simulink model "EPT"  (R2019b)
settings: Solver=FixedStepDiscrete  StartTime=0.0  StopTime=5  FixedStep=0.005  RelTol=1e-3  EnableMultiTasking=on
PreLoadFcn:
  | try, model_open; catch, disp('Error occurred while executing model pre-load callback: model_open.m'); disp('Please assure that the MATLAB working directory is set to the model directory before opening.'); end
InitFcn:
  | try, model_open; catch, end
undefined symbols (not defined in the file or in its folder): Bridge, GCM, H, ln, raptor_get_param_eval, raptor_get_safe_string, raptor_xcp_function
libraries: Raptor_lib x2810, simulink x374, hdlsllib x19
(part 7 of 45)

== system EPT/I//O/Output/DualLED_Half_Bridge ==
  note: H3
  note: H1
  Data Type Conversion : DataTypeConversion
  Data Type Conversion3 : DataTypeConversion
  Gain : Gain  Gain=100
  Gain3 : Gain  Gain=100
  raptor_adjustment1 : Raptor_lib/Data Storage/raptor_adjustment  paramName='A43_A44_HalfBridge_Brake'  nameSource=Parameter  initValue=0.00  dataType=boolean  storage=Calibration  calDispType=Number  calEnum={'False', 'True'}  calGain=1.0  calOffset=0.0  calMax=inf  calMin=-inf  calFormat='-1'  calUnit=''  calHelp=''  calAccess=1  calFunction=raptor_xcp_function(gcb)  calDispHeaders=off  calColHeaders={'Col1' 'Col2' 'Col3'}  calRowHeaders={'Row1' 'Row2' 'Row3'}
      settings: SourceProductName=Raptor
  raptor_adjustment2 : Raptor_lib/Data Storage/raptor_adjustment  paramName='Cal_HalfBridge3_Freq'  nameSource=Parameter  initValue=1000  dataType=uint16  storage=Calibration  calDispType=Number  calEnum={'False', 'True'}  calGain=1.0  calOffset=0.0  calMax=inf  calMin=-inf  calFormat='-1'  calUnit=''  calHelp=''  calAccess=1  calFunction=raptor_xcp_function(gcb)  calDispHeaders=off  calColHeaders={'Col1' 'Col2' 'Col3'}  calRowHeaders={'Row1' 'Row2' 'Row3'}
      settings: SourceProductName=Raptor
  raptor_adjustment3 : Raptor_lib/Data Storage/raptor_adjustment  paramName='Cal_HalfBridge3_En'  nameSource=Parameter  initValue=1  dataType=boolean  storage=Calibration  calDispType=Number  calEnum={'False', 'True'}  calGain=1.0  calOffset=0.0  calMax=inf  calMin=-inf  calFormat='-1'  calUnit=''  calHelp=''  calAccess=1  calFunction=raptor_xcp_function(gcb)  calDispHeaders=off  calColHeaders={'Col1' 'Col2' 'Col3'}  calRowHeaders={'Row1' 'Row2' 'Row3'}
      settings: SourceProductName=Raptor
  raptor_adjustment4 : Raptor_lib/Data Storage/raptor_adjustment  paramName='A66_A67_HalfBridge_Brake'  nameSource=Parameter  initValue=0.00  dataType=boolean  storage=Calibration  calDispType=Number  calEnum={'False', 'True'}  calGain=1.0  calOffset=0.0  calMax=inf  calMin=-inf  calFormat='-1'  calUnit=''  calHelp=''  calAccess=1  calFunction=raptor_xcp_function(gcb)  calDispHeaders=off  calColHeaders={'Col1' 'Col2' 'Col3'}  calRowHeaders={'Row1' 'Row2' 'Row3'}
      settings: SourceProductName=Raptor
  raptor_adjustment5 : Raptor_lib/Data Storage/raptor_adjustment  paramName='Cal_HalfBridge1_Freq'  nameSource=Parameter  initValue=1000  dataType=uint16  storage=Calibration  calDispType=Number  calEnum={'False', 'True'}  calGain=1.0  calOffset=0.0  calMax=inf  calMin=-inf  calFormat='-1'  calUnit=''  calHelp=''  calAccess=1  calFunction=raptor_xcp_function(gcb)  calDispHeaders=off  calColHeaders={'Col1' 'Col2' 'Col3'}  calRowHeaders={'Row1' 'Row2' 'Row3'}
      settings: SourceProductName=Raptor
  raptor_adjustment6 : Raptor_lib/Data Storage/raptor_adjustment  paramName='Cal_HalfBridge1_En'  nameSource=Parameter  initValue=1  dataType=boolean  storage=Calibration  calDispType=Number  calEnum={'False', 'True'}  calGain=1.0  calOffset=0.0  calMax=inf  calMin=-inf  calFormat='-1'  calUnit=''  calHelp=''  calAccess=1  calFunction=raptor_xcp_function(gcb)  calDispHeaders=off  calColHeaders={'Col1' 'Col2' 'Col3'}  calRowHeaders={'Row1' 'Row2' 'Row3'}
      settings: SourceProductName=Raptor
  raptor_data_read : Raptor_lib/Data Storage/raptor_data_read  dataName='LED_Duty'  dataShape=Scalar  idxSource=Input  idxRow=1  idxCol=1
      settings: SourceProductName=Raptor
  raptor_hbridge_out : Raptor_lib/Input & Output/raptor_hbridge_out  resourceValues=OUTPUT50_51|OUTPUT52_53|OUTPUT54_55|(None)  resource=OUTPUT54_55  outError=0  driverTypeValues=H-Bridge  driverType=H-Bridge
      settings: SourceProductName=Raptor
  raptor_hbridge_out1 : Raptor_lib/Input & Output/raptor_hbridge_out  resourceValues=OUTPUT50_51|OUTPUT52_53|OUTPUT54_55|(None)  resource=OUTPUT50_51  outError=0  driverTypeValues=H-Bridge  driverType=H-Bridge
      settings: SourceProductName=Raptor
  wires:
  raptor_adjustment1/1 -> raptor_hbridge_out/2
  raptor_data_read/1 -> raptor_hbridge_out1/3, raptor_hbridge_out/3
  Gain/1 -> Data Type Conversion/1
  Data Type Conversion/1 -> raptor_hbridge_out/4
  raptor_adjustment3/1 -> raptor_hbridge_out/1
  raptor_adjustment2/1 -> Gain/1
  raptor_adjustment4/1 -> raptor_hbridge_out1/2
  raptor_adjustment5/1 -> Gain3/1
  Data Type Conversion3/1 -> raptor_hbridge_out1/4
  Gain3/1 -> Data Type Conversion3/1
  raptor_adjustment6/1 -> raptor_hbridge_out1/1

== system EPT/I//O/Output/Lamp_Sound ==
  raptor_adjustment : Raptor_lib/Data Storage/raptor_adjustment  paramName='A01_LSD_EW_Sound1'  nameSource=Parameter  initValue=0.00  dataType=boolean  storage=Calibration  calDispType=Number  calEnum={'False', 'True'}  calGain=1.0  calOffset=0.0  calMax=inf  calMin=-inf  calFormat='-1'  calUnit=''  calHelp=''  calAccess=1  calFunction=raptor_xcp_function(gcb)  calDispHeaders=off  calColHeaders={'Col1' 'Col2' 'Col3'}  calRowHeaders={'Row1' 'Row2' 'Row3'}
      settings: SourceProductName=Raptor
  raptor_adjustment3 : Raptor_lib/Data Storage/raptor_adjustment  paramName='A54_EW_Lamp_Sound3'  nameSource=Parameter  initValue=0.00  dataType=boolean  storage=Calibration  calDispType=Number  calEnum={'False', 'True'}  calGain=1.0  calOffset=0.0  calMax=inf  calMin=-inf  calFormat='-1'  calUnit=''  calHelp=''  calAccess=1  calFunction=raptor_xcp_function(gcb)  calDispHeaders=off  calColHeaders={'Col1' 'Col2' 'Col3'}  calRowHeaders={'Row1' 'Row2' 'Row3'}
      settings: SourceProductName=Raptor
  raptor_digital_out : Raptor_lib/Input & Output/raptor_digital_out  resourceValues=OUTPUT1|OUTPUT2|OUTPUT3|OUTPUT4|OUTPUT5|OUTPUT6|OUTPUT7|OUTPUT8|OUTPUT9|OUTPUT10|OUTPUT11|OUTPUT12|OUTPUT21|OUTPUT22|OUTPUT23|OUTPUT24|OUTPUT25|OUTPUT26|OUTPUT27|OUTPUT28|OUTPUT29|OUTPUT30|OUTPUT31|OUTPUT32|OUTPUT33|OUTPUT34|OUTPUT35|OUTPUT36|OUTPUT37|OUTPUT38|OUTPUT39|OUTPUT40|OUTPUT41|OUTPUT42|OUTPUT43|OUTPUT44|OUTPUT45|OUTPUT46|OUTPUT47|OUTPUT48|OUTPUT49|POWER_HOLD|(None)  resource=OUTPUT25  driverTypeValues=Low Side  driverType=Low Side
      settings: SourceProductName=Raptor
  raptor_digital_out3 : Raptor_lib/Input & Output/raptor_digital_out  resourceValues=OUTPUT1|OUTPUT2|OUTPUT3|OUTPUT4|OUTPUT5|OUTPUT6|OUTPUT7|OUTPUT8|OUTPUT9|OUTPUT10|OUTPUT11|OUTPUT12|OUTPUT21|OUTPUT22|OUTPUT23|OUTPUT24|OUTPUT25|OUTPUT26|OUTPUT27|OUTPUT28|OUTPUT29|OUTPUT30|OUTPUT31|OUTPUT32|OUTPUT33|OUTPUT34|OUTPUT35|OUTPUT36|OUTPUT37|OUTPUT38|OUTPUT39|OUTPUT40|OUTPUT41|OUTPUT42|OUTPUT43|OUTPUT44|OUTPUT45|OUTPUT46|OUTPUT47|OUTPUT48|OUTPUT49|POWER_HOLD|(None)  resource=OUTPUT5  driverTypeValues=Low Side  driverType=Low Side
      settings: SourceProductName=Raptor
  wires:
  raptor_adjustment3/1 -> raptor_digital_out3/1
  raptor_adjustment/1 -> raptor_digital_out/1

== system EPT/I//O/Output/RelayBox ==
  Bitwe Operator{2..7} (6 alike) : simulink/Logic and Bit Operations/Bitwise Operator  logicop=OR  UseBitMask=off  NumInputPorts=2  BitMask=bin2dec('11011001')  BitMaskRealWorld=Stored Integer
  raptor_adjustment : Raptor_lib/Data Storage/raptor_adjustment  paramName='K12_LSD_Relay_HV_Body'  nameSource=Parameter  initValue=0.00  dataType=boolean  storage=Calibration  calDispType=Number  calEnum={'False', 'True'}  calGain=1.0  calOffset=0.0  calMax=inf  calMin=-inf  calFormat='-1'  calUnit=''  calHelp=''  calAccess=1  calFunction=raptor_xcp_function(gcb)  calDispHeaders=off  calColHeaders={'Col1' 'Col2' 'Col3'}  calRowHeaders={'Row1' 'Row2' 'Row3'}
      settings: SourceProductName=Raptor
  raptor_adjustment2 : Raptor_lib/Data Storage/raptor_adjustment  paramName='K20_LSD_Relay_DCDC_12V'  nameSource=Parameter  initValue=0.00  dataType=boolean  storage=Calibration  calDispType=Number  calEnum={'False', 'True'}  calGain=1.0  calOffset=0.0  calMax=inf  calMin=-inf  calFormat='-1'  calUnit=''  calHelp=''  calAccess=1  calFunction=raptor_xcp_function(gcb)  calDispHeaders=off  calColHeaders={'Col1' 'Col2' 'Col3'}  calRowHeaders={'Row1' 'Row2' 'Row3'}
      settings: SourceProductName=Raptor
  raptor_adjustment3 : Raptor_lib/Data Storage/raptor_adjustment  paramName='K36_LSD_Relay_CHG_OBC'  nameSource=Parameter  initValue=0.00  dataType=boolean  storage=Calibration  calDispType=Number  calEnum={'False', 'True'}  calGain=1.0  calOffset=0.0  calMax=inf  calMin=-inf  calFormat='-1'  calUnit=''  calHelp=''  calAccess=1  calFunction=raptor_xcp_function(gcb)  calDispHeaders=off  calColHeaders={'Col1' 'Col2' 'Col3'}  calRowHeaders={'Row1' 'Row2' 'Row3'}
      settings: SourceProductName=Raptor
  raptor_adjustment4 : Raptor_lib/Data Storage/raptor_adjustment  paramName='K38_LSD_Relay_BMS_OBU'  nameSource=Parameter  initValue=0.00  dataType=boolean  storage=Calibration  calDispType=Number  calEnum={'False', 'True'}  calGain=1.0  calOffset=0.0  calMax=inf  calMin=-inf  calFormat='-1'  calUnit=''  calHelp=''  calAccess=1  calFunction=raptor_xcp_function(gcb)  calDispHeaders=off  calColHeaders={'Col1' 'Col2' 'Col3'}  calRowHeaders={'Row1' 'Row2' 'Row3'}
      settings: SourceProductName=Raptor
  raptor_adjustment5 : Raptor_lib/Data Storage/raptor_adjustment  paramName='K39_LSD_Relay_MCU'  nameSource=Parameter  initValue=0.00  dataType=boolean  storage=Calibration  calDispType=Number  calEnum={'False', 'True'}  calGain=1.0  calOffset=0.0  calMax=inf  calMin=-inf  calFormat='-1'  calUnit=''  calHelp=''  calAccess=1  calFunction=raptor_xcp_function(gcb)  calDispHeaders=off  calColHeaders={'Col1' 'Col2' 'Col3'}  calRowHeaders={'Row1' 'Row2' 'Row3'}
      settings: SourceProductName=Raptor
  raptor_adjustment6 : Raptor_lib/Data Storage/raptor_adjustment  paramName='K56_LSD_Relay_BMS_SWU'  nameSource=Parameter  initValue=0.00  dataType=boolean  storage=Calibration  calDispType=Number  calEnum={'False', 'True'}  calGain=1.0  calOffset=0.0  calMax=inf  calMin=-inf  calFormat='-1'  calUnit=''  calHelp=''  calAccess=1  calFunction=raptor_xcp_function(gcb)  calDispHeaders=off  calColHeaders={'Col1' 'Col2' 'Col3'}  calRowHeaders={'Row1' 'Row2' 'Row3'}
      settings: SourceProductName=Raptor
  raptor_data_def : Raptor_lib/Data Storage/raptor_data_def  dataName='Relay_HV_Body'  initValue=0  dataType=boolean  storage=Volatile (RAM)  calVisible=on  calType=Measurement  calDispType=Number  calEnum={'False', 'True'}  calGain=1.0  calOffset=0  calMin=-inf  calMax=inf  calFormat='-1'  calUnit=''  calHelp=''  calAccess=1  calFunction=raptor_xcp_function(gcb)  calDispHeaders=off  calColHeaders={'Col1' 'Col2' 'Col3'}  calRowHeaders={'Row1' 'Row2' 'Row3'}
      settings: SourceProductName=Raptor
  raptor_data_def2 : Raptor_lib/Data Storage/raptor_data_def  dataName='Relay_DCDC_12V'  initValue=0  dataType=boolean  storage=Volatile (RAM)  calVisible=on  calType=Measurement  calDispType=Number  calEnum={'False', 'True'}  calGain=1.0  calOffset=0  calMin=-inf  calMax=inf  calFormat='-1'  calUnit=''  calHelp=''  calAccess=1  calFunction=raptor_xcp_function(gcb)  calDispHeaders=off  calColHeaders={'Col1' 'Col2' 'Col3'}  calRowHeaders={'Row1' 'Row2' 'Row3'}
      settings: SourceProductName=Raptor
  raptor_data_def3 : Raptor_lib/Data Storage/raptor_data_def  dataName='Relay_CHG_OBC'  initValue=0  dataType=boolean  storage=Volatile (RAM)  calVisible=on  calType=Measurement  calDispType=Number  calEnum={'False', 'True'}  calGain=1.0  calOffset=0  calMin=-inf  calMax=inf  calFormat='-1'  calUnit=''  calHelp=''  calAccess=1  calFunction=raptor_xcp_function(gcb)  calDispHeaders=off  calColHeaders={'Col1' 'Col2' 'Col3'}  calRowHeaders={'Row1' 'Row2' 'Row3'}
      settings: SourceProductName=Raptor
  raptor_data_def4 : Raptor_lib/Data Storage/raptor_data_def  dataName='Relay_BMS_OBU'  initValue=0  dataType=boolean  storage=Volatile (RAM)  calVisible=on  calType=Measurement  calDispType=Number  calEnum={'False', 'True'}  calGain=1.0  calOffset=0  calMin=-inf  calMax=inf  calFormat='-1'  calUnit=''  calHelp=''  calAccess=1  calFunction=raptor_xcp_function(gcb)  calDispHeaders=off  calColHeaders={'Col1' 'Col2' 'Col3'}  calRowHeaders={'Row1' 'Row2' 'Row3'}
      settings: SourceProductName=Raptor
  raptor_data_def5 : Raptor_lib/Data Storage/raptor_data_def  dataName='Relay_MCU'  initValue=0  dataType=boolean  storage=Volatile (RAM)  calVisible=on  calType=Measurement  calDispType=Number  calEnum={'False', 'True'}  calGain=1.0  calOffset=0  calMin=-inf  calMax=inf  calFormat='-1'  calUnit=''  calHelp=''  calAccess=1  calFunction=raptor_xcp_function(gcb)  calDispHeaders=off  calColHeaders={'Col1' 'Col2' 'Col3'}  calRowHeaders={'Row1' 'Row2' 'Row3'}
      settings: SourceProductName=Raptor
  raptor_data_def6 : Raptor_lib/Data Storage/raptor_data_def  dataName='Relay_BMS_SWU'  initValue=0  dataType=boolean  storage=Volatile (RAM)  calVisible=on  calType=Measurement  calDispType=Number  calEnum={'False', 'True'}  calGain=1.0  calOffset=0  calMin=-inf  calMax=inf  calFormat='-1'  calUnit=''  calHelp=''  calAccess=1  calFunction=raptor_xcp_function(gcb)  calDispHeaders=off  calColHeaders={'Col1' 'Col2' 'Col3'}  calRowHeaders={'Row1' 'Row2' 'Row3'}
      settings: SourceProductName=Raptor
  raptor_data_read : Raptor_lib/Data Storage/raptor_data_read  dataName='Relay_BMS_OBU'  dataShape=Scalar  idxSource=Input  idxRow=1  idxCol=1
      settings: SourceProductName=Raptor
  raptor_data_read1 : Raptor_lib/Data Storage/raptor_data_read  dataName='Relay_MCU'  dataShape=Scalar  idxSource=Input  idxRow=1  idxCol=1
      settings: SourceProductName=Raptor
  raptor_data_read2 : Raptor_lib/Data Storage/raptor_data_read  dataName='Relay_BMS_SWU'  dataShape=Scalar  idxSource=Input  idxRow=1  idxCol=1
      settings: SourceProductName=Raptor
  raptor_data_read4 : Raptor_lib/Data Storage/raptor_data_read  dataName='Relay_CHG_OBC'  dataShape=Scalar  idxSource=Input  idxRow=1  idxCol=1
      settings: SourceProductName=Raptor
  raptor_data_read5 : Raptor_lib/Data Storage/raptor_data_read  dataName='Relay_DCDC_12V'  dataShape=Scalar  idxSource=Input  idxRow=1  idxCol=1
      settings: SourceProductName=Raptor
  raptor_data_read7 : Raptor_lib/Data Storage/raptor_data_read  dataName='Relay_HV_Body'  dataShape=Scalar  idxSource=Input  idxRow=1  idxCol=1
      settings: SourceProductName=Raptor
  raptor_digital_out : Raptor_lib/Input & Output/raptor_digital_out  resourceValues=OUTPUT1|OUTPUT2|OUTPUT3|OUTPUT4|OUTPUT5|OUTPUT6|OUTPUT7|OUTPUT8|OUTPUT9|OUTPUT10|OUTPUT11|OUTPUT12|OUTPUT21|OUTPUT22|OUTPUT23|OUTPUT24|OUTPUT25|OUTPUT26|OUTPUT27|OUTPUT28|OUTPUT29|OUTPUT30|OUTPUT31|OUTPUT32|OUTPUT33|OUTPUT34|OUTPUT35|OUTPUT36|OUTPUT37|OUTPUT38|OUTPUT39|OUTPUT40|OUTPUT41|OUTPUT42|OUTPUT43|OUTPUT44|OUTPUT45|OUTPUT46|OUTPUT47|OUTPUT48|OUTPUT49|POWER_HOLD|(None)  resource=OUTPUT33  driverTypeValues=Low Side  driverType=Low Side
      settings: SourceProductName=Raptor
  raptor_digital_out2 : Raptor_lib/Input & Output/raptor_digital_out  resourceValues=OUTPUT1|OUTPUT2|OUTPUT3|OUTPUT4|OUTPUT5|OUTPUT6|OUTPUT7|OUTPUT8|OUTPUT9|OUTPUT10|OUTPUT11|OUTPUT12|OUTPUT21|OUTPUT22|OUTPUT23|OUTPUT24|OUTPUT25|OUTPUT26|OUTPUT27|OUTPUT28|OUTPUT29|OUTPUT30|OUTPUT31|OUTPUT32|OUTPUT33|OUTPUT34|OUTPUT35|OUTPUT36|OUTPUT37|OUTPUT38|OUTPUT39|OUTPUT40|OUTPUT41|OUTPUT42|OUTPUT43|OUTPUT44|OUTPUT45|OUTPUT46|OUTPUT47|OUTPUT48|OUTPUT49|POWER_HOLD|(None)  resource=OUTPUT35  driverTypeValues=Low Side  driverType=Low Side
      settings: SourceProductName=Raptor
  raptor_digital_out3 : Raptor_lib/Input & Output/raptor_digital_out  resourceValues=OUTPUT1|OUTPUT2|OUTPUT3|OUTPUT4|OUTPUT5|OUTPUT6|OUTPUT7|OUTPUT8|OUTPUT9|OUTPUT10|OUTPUT11|OUTPUT12|OUTPUT21|OUTPUT22|OUTPUT23|OUTPUT24|OUTPUT25|OUTPUT26|OUTPUT27|OUTPUT28|OUTPUT29|OUTPUT30|OUTPUT31|OUTPUT32|OUTPUT33|OUTPUT34|OUTPUT35|OUTPUT36|OUTPUT37|OUTPUT38|OUTPUT39|OUTPUT40|OUTPUT41|OUTPUT42|OUTPUT43|OUTPUT44|OUTPUT45|OUTPUT46|OUTPUT47|OUTPUT48|OUTPUT49|POWER_HOLD|(None)  resource=OUTPUT37  driverTypeValues=Low Side  driverType=Low Side
      settings: SourceProductName=Raptor
  raptor_digital_out4 : Raptor_lib/Input & Output/raptor_digital_out  resourceValues=OUTPUT1|OUTPUT2|OUTPUT3|OUTPUT4|OUTPUT5|OUTPUT6|OUTPUT7|OUTPUT8|OUTPUT9|OUTPUT10|OUTPUT11|OUTPUT12|OUTPUT21|OUTPUT22|OUTPUT23|OUTPUT24|OUTPUT25|OUTPUT26|OUTPUT27|OUTPUT28|OUTPUT29|OUTPUT30|OUTPUT31|OUTPUT32|OUTPUT33|OUTPUT34|OUTPUT35|OUTPUT36|OUTPUT37|OUTPUT38|OUTPUT39|OUTPUT40|OUTPUT41|OUTPUT42|OUTPUT43|OUTPUT44|OUTPUT45|OUTPUT46|OUTPUT47|OUTPUT48|OUTPUT49|POWER_HOLD|(None)  resource=OUTPUT38  driverTypeValues=Low Side  driverType=Low Side
      settings: SourceProductName=Raptor
  raptor_digital_out5 : Raptor_lib/Input & Output/raptor_digital_out  resourceValues=OUTPUT1|OUTPUT2|OUTPUT3|OUTPUT4|OUTPUT5|OUTPUT6|OUTPUT7|OUTPUT8|OUTPUT9|OUTPUT10|OUTPUT11|OUTPUT12|OUTPUT21|OUTPUT22|OUTPUT23|OUTPUT24|OUTPUT25|OUTPUT26|OUTPUT27|OUTPUT28|OUTPUT29|OUTPUT30|OUTPUT31|OUTPUT32|OUTPUT33|OUTPUT34|OUTPUT35|OUTPUT36|OUTPUT37|OUTPUT38|OUTPUT39|OUTPUT40|OUTPUT41|OUTPUT42|OUTPUT43|OUTPUT44|OUTPUT45|OUTPUT46|OUTPUT47|OUTPUT48|OUTPUT49|POWER_HOLD|(None)  resource=OUTPUT39  driverTypeValues=Low Side  driverType=Low Side
      settings: SourceProductName=Raptor
  raptor_digital_out6 : Raptor_lib/Input & Output/raptor_digital_out  resourceValues=OUTPUT1|OUTPUT2|OUTPUT3|OUTPUT4|OUTPUT5|OUTPUT6|OUTPUT7|OUTPUT8|OUTPUT9|OUTPUT10|OUTPUT11|OUTPUT12|OUTPUT21|OUTPUT22|OUTPUT23|OUTPUT24|OUTPUT25|OUTPUT26|OUTPUT27|OUTPUT28|OUTPUT29|OUTPUT30|OUTPUT31|OUTPUT32|OUTPUT33|OUTPUT34|OUTPUT35|OUTPUT36|OUTPUT37|OUTPUT38|OUTPUT39|OUTPUT40|OUTPUT41|OUTPUT42|OUTPUT43|OUTPUT44|OUTPUT45|OUTPUT46|OUTPUT47|OUTPUT48|OUTPUT49|POWER_HOLD|(None)  resource=OUTPUT42  driverTypeValues=Low Side  driverType=Low Side
      settings: SourceProductName=Raptor
  raptor_override : Raptor_lib/Data Storage/raptor_override  paramName='Cal_Relay_DCDC_12V'  nameSource=Parameter  measurement=None  calDispType=Number  calEnum={'False', 'True'}  calGain=1.0  calOffset=0.0  calMax=inf  calMin=-inf  calFormat='-1'  calUnit=''  calHelp=''  calAccess=1  calFunction=[raptor_xcp_function(gcb) '|' raptor_get_param_eval(gcb, 'paramName') '_Override']
      settings: SourceProductName=Raptor
  raptor_override1 : Raptor_lib/Data Storage/raptor_override  paramName='Cal_Relay_HV_Body'  nameSource=Parameter  measurement=None  calDispType=Number  calEnum={'False', 'True'}  calGain=1.0  calOffset=0.0  calMax=inf  calMin=-inf  calFormat='-1'  calUnit=''  calHelp=''  calAccess=1  calFunction=[raptor_xcp_function(gcb) '|' raptor_get_param_eval(gcb, 'paramName') '_Override']
      settings: SourceProductName=Raptor
  raptor_override2 : Raptor_lib/Data Storage/raptor_override  paramName='Cal_Relay_CHG_OBC'  nameSource=Parameter  measurement=None  calDispType=Number  calEnum={'False', 'True'}  calGain=1.0  calOffset=0.0  calMax=inf  calMin=-inf  calFormat='-1'  calUnit=''  calHelp=''  calAccess=1  calFunction=[raptor_xcp_function(gcb) '|' raptor_get_param_eval(gcb, 'paramName') '_Override']
      settings: SourceProductName=Raptor
  raptor_override3 : Raptor_lib/Data Storage/raptor_override  paramName='Cal_Relay_BMS_OBU'  nameSource=Parameter  measurement=None  calDispType=Number  calEnum={'False', 'True'}  calGain=1.0  calOffset=0.0  calMax=inf  calMin=-inf  calFormat='-1'  calUnit=''  calHelp=''  calAccess=1  calFunction=[raptor_xcp_function(gcb) '|' raptor_get_param_eval(gcb, 'paramName') '_Override']
      settings: SourceProductName=Raptor
  raptor_override4 : Raptor_lib/Data Storage/raptor_override  paramName='Cal_Relay_MCU'  nameSource=Parameter  measurement=None  calDispType=Number  calEnum={'False', 'True'}  calGain=1.0  calOffset=0.0  calMax=inf  calMin=-inf  calFormat='-1'  calUnit=''  calHelp=''  calAccess=1  calFunction=[raptor_xcp_function(gcb) '|' raptor_get_param_eval(gcb, 'paramName') '_Override']
      settings: SourceProductName=Raptor
  raptor_override5 : Raptor_lib/Data Storage/raptor_override  paramName='Cal_Relay_BMS_SWU'  nameSource=Parameter  measurement=None  calDispType=Number  calEnum={'False', 'True'}  calGain=1.0  calOffset=0.0  calMax=inf  calMin=-inf  calFormat='-1'  calUnit=''  calHelp=''  calAccess=1  calFunction=[raptor_xcp_function(gcb) '|' raptor_get_param_eval(gcb, 'paramName') '_Override']
      settings: SourceProductName=Raptor
  wires:
  raptor_adjustment/1 -> Bitwe Operator5/1
  raptor_adjustment2/1 -> Bitwe Operator2/1
  raptor_adjustment3/1 -> Bitwe Operator3/1
  raptor_adjustment4/1 -> Bitwe Operator4/1
  raptor_adjustment5/1 -> Bitwe Operator6/1
  raptor_adjustment6/1 -> Bitwe Operator7/1
  raptor_data_read2/1 -> Bitwe Operator7/2
  Bitwe Operator7/1 -> raptor_override5/1
  Bitwe Operator6/1 -> raptor_override4/1
  raptor_data_read1/1 -> Bitwe Operator6/2
  Bitwe Operator4/1 -> raptor_override3/1
  raptor_data_read/1 -> Bitwe Operator4/2
  raptor_data_read4/1 -> Bitwe Operator3/2
  Bitwe Operator3/1 -> raptor_override2/1
  raptor_data_read5/1 -> Bitwe Operator2/2
  Bitwe Operator2/1 -> raptor_override/1
  Bitwe Operator5/1 -> raptor_override1/1
  raptor_data_read7/1 -> Bitwe Operator5/2
  raptor_override/1 -> raptor_digital_out2/1
  raptor_override1/1 -> raptor_digital_out/1
  raptor_override2/1 -> raptor_digital_out3/1
  raptor_override3/1 -> raptor_digital_out4/1
  raptor_override4/1 -> raptor_digital_out5/1
  raptor_override5/1 -> raptor_digital_out6/1

== system EPT/I//O/Output/Reserved ==
  raptor_adjustment1 : Raptor_lib/Data Storage/raptor_adjustment  paramName='K84_LSD_PWM_Reserved1'  nameSource=Parameter  initValue=0.00  dataType=boolean  storage=Calibration  calDispType=Number  calEnum={'False', 'True'}  calGain=1.0  calOffset=0.0  calMax=inf  calMin=-inf  calFormat='-1'  calUnit=''  calHelp=''  calAccess=1  calFunction=raptor_xcp_function(gcb)  calDispHeaders=off  calColHeaders={'Col1' 'Col2' 'Col3'}  calRowHeaders={'Row1' 'Row2' 'Row3'}
      settings: SourceProductName=Raptor
  raptor_data_def : Raptor_lib/Data Storage/raptor_data_def  dataName='K57_LSD_WakeUp_Reserved'  initValue=0  dataType=boolean  storage=Calibration  calVisible=on  calType=Measurement  calDispType=Number  calEnum={'False', 'True'}  calGain=1.0  calOffset=0  calMin=-inf  calMax=inf  calFormat='-1'  calUnit=''  calHelp=''  calAccess=1  calFunction=raptor_xcp_function(gcb)  calDispHeaders=off  calColHeaders={'Col1' 'Col2' 'Col3'}  calRowHeaders={'Row1' 'Row2' 'Row3'}
      settings: SourceProductName=Raptor
  raptor_data_read : Raptor_lib/Data Storage/raptor_data_read  dataName='K57_LSD_WakeUp_Reserved'  dataShape=Scalar  idxSource=Input  idxRow=1  idxCol=1
      settings: SourceProductName=Raptor
  raptor_digital_out1 : Raptor_lib/Input & Output/raptor_digital_out  resourceValues=OUTPUT1|OUTPUT2|OUTPUT3|OUTPUT4|OUTPUT5|OUTPUT6|OUTPUT7|OUTPUT8|OUTPUT9|OUTPUT10|OUTPUT11|OUTPUT12|OUTPUT21|OUTPUT22|OUTPUT23|OUTPUT24|OUTPUT25|OUTPUT26|OUTPUT27|OUTPUT28|OUTPUT29|OUTPUT30|OUTPUT31|OUTPUT32|OUTPUT33|OUTPUT34|OUTPUT35|OUTPUT36|OUTPUT37|OUTPUT38|OUTPUT39|OUTPUT40|OUTPUT41|OUTPUT42|OUTPUT43|OUTPUT44|OUTPUT45|OUTPUT46|OUTPUT47|OUTPUT48|OUTPUT49|POWER_HOLD|(None)  resource=OUTPUT7  driverTypeValues=Low Side  driverType=Low Side
      settings: SourceProductName=Raptor
  raptor_digital_out2 : Raptor_lib/Input & Output/raptor_digital_out  resourceValues=OUTPUT1|OUTPUT2|OUTPUT3|OUTPUT4|OUTPUT5|OUTPUT6|OUTPUT7|OUTPUT8|OUTPUT9|OUTPUT10|OUTPUT11|OUTPUT12|OUTPUT21|OUTPUT22|OUTPUT23|OUTPUT24|OUTPUT25|OUTPUT26|OUTPUT27|OUTPUT28|OUTPUT29|OUTPUT30|OUTPUT31|OUTPUT32|OUTPUT33|OUTPUT34|OUTPUT35|OUTPUT36|OUTPUT37|OUTPUT38|OUTPUT39|OUTPUT40|OUTPUT41|OUTPUT42|OUTPUT43|OUTPUT44|OUTPUT45|OUTPUT46|OUTPUT47|OUTPUT48|OUTPUT49|POWER_HOLD|(None)  resource=OUTPUT11  driverTypeValues=Low Side  driverType=Low Side
      settings: SourceProductName=Raptor
  wires:
  raptor_adjustment1/1 -> raptor_digital_out1/1
  raptor_data_read/1 -> raptor_digital_out2/1

== system EPT/LED_Status/DualLED_Funny/LED_Status ==
  0.5Hz : Subsystem  TreatAsAtomicUnit=on
  100Hz : Subsystem  TreatAsAtomicUnit=on
  10Hz : Subsystem  TreatAsAtomicUnit=on
  1Hz : Subsystem  TreatAsAtomicUnit=on
  2Hz : Subsystem  TreatAsAtomicUnit=on
  4Hz : Subsystem  TreatAsAtomicUnit=on
  Alarrn_LED : Subsystem  TreatAsAtomicUnit=on
  Charging : Subsystem  TreatAsAtomicUnit=on
  Constant1 : Constant  Value=100
  Constant10 : Constant  Value=5
  Constant11 : Constant  Value=6
  Constant12 : Constant
  Constant13 : Constant  Value=0
  Constant2 : Constant  Value=200
  Constant3 : Constant  Value=10
  Constant4 : Constant  Value=50
  Constant5 : Constant  Value=25
  Constant7 : Constant  Value=7
  Constant8 : Constant  Value=3
  Constant9 : Constant  Value=4
  CountTrigger1 : Subsystem
  CountTrigger2 : Subsystem
  CountTrigger3 : Subsystem
  CountTrigger4 : Subsystem
  CountTrigger5 : Subsystem
  CountTrigger6 : Subsystem
  "D " : Subsystem  TreatAsAtomicUnit=on
  EVSE Conected : Subsystem  TreatAsAtomicUnit=on
  Logical Operator{,1..3,5} (5 alike) : Logic  AllPortsSameDT=off  OutDataTypeStr=boolean
  Logical Operator4 : Logic  Operator=OR  AllPortsSameDT=off  OutDataTypeStr=boolean
  N : Subsystem  TreatAsAtomicUnit=on
  NOT : Logic  Operator=NOT  IconShape=distinctive  AllPortsSameDT=off  OutDataTypeStr=boolean
  NOT1 : Logic  Operator=NOT  IconShape=distinctive  AllPortsSameDT=off  OutDataTypeStr=boolean
  No Mode : Subsystem  TreatAsAtomicUnit=on
  P : Subsystem  TreatAsAtomicUnit=on
  R : Subsystem  TreatAsAtomicUnit=on
  Switch{,1..6} (7 alike) : Switch  Criteria=u2 > Threshold
  Switch Case : SwitchCase  CaseConditions={0,1,2,3,4,5,6,7}  ShowDefaultCase=off
  raptor_adjustment : Raptor_lib/Data Storage/raptor_adjustment  paramName='Cal_No_Mode_Freq'  nameSource=Parameter  initValue=2  dataType=double  storage=Calibration  calDispType=Number  calEnum={'False', 'True'}  calGain=1.0  calOffset=0.0  calMax=inf  calMin=-inf  calFormat='-1'  calUnit=''  calHelp=''  calAccess=1  calFunction=raptor_xcp_function(gcb)  calDispHeaders=off  calColHeaders={'Col1' 'Col2' 'Col3'}  calRowHeaders={'Row1' 'Row2' 'Row3'}
      settings: SourceProductName=Raptor
  raptor_data_def : Raptor_lib/Data Storage/raptor_data_def  dataName='LED_Duty'  initValue=0  dataType=int16  storage=Volatile (RAM)  calVisible=on  calType=Measurement  calDispType=Number  calEnum={'False', 'True'}  calGain=1.0  calOffset=0  calMin=-inf  calMax=inf  calFormat='-1'  calUnit=''  calHelp=''  calAccess=1  calFunction=raptor_xcp_function(gcb)  calDispHeaders=off  calColHeaders={'Col1' 'Col2' 'Col3'}  calRowHeaders={'Row1' 'Row2' 'Row3'}
      settings: SourceProductName=Raptor
  raptor_data_def1 : Raptor_lib/Data Storage/raptor_data_def  dataName='LED_Gradient'  initValue=0  dataType=boolean  storage=Volatile (RAM)  calVisible=on  calType=Measurement  calDispType=Number  calEnum={'False', 'True'}  calGain=1.0  calOffset=0  calMin=-inf  calMax=inf  calFormat='-1'  calUnit=''  calHelp=''  calAccess=1  calFunction=raptor_xcp_function(gcb)  calDispHeaders=off  calColHeaders={'Col1' 'Col2' 'Col3'}  calRowHeaders={'Row1' 'Row2' 'Row3'}
      settings: SourceProductName=Raptor
  raptor_data_def51 : Raptor_lib/Data Storage/raptor_data_def  dataName='LED_Status'  initValue=0  dataType=uint8  storage=Volatile (RAM)  calVisible=on  calType=Measurement  calDispType=Number  calEnum={'False', 'True'}  calGain=1.0  calOffset=0  calMin=-inf  calMax=inf  calFormat='-1'  calUnit=''  calHelp=''  calAccess=1  calFunction=raptor_xcp_function(gcb)  calDispHeaders=off  calColHeaders={'Col1' 'Col2' 'Col3'}  calRowHeaders={'Row1' 'Row2' 'Row3'}
      settings: SourceProductName=Raptor
  raptor_data_read1 : Raptor_lib/Data Storage/raptor_data_read  dataName='LED_Status'  dataShape=Scalar  idxSource=Input  idxRow=1  idxCol=1
      settings: SourceProductName=Raptor
  raptor_data_read2 : Raptor_lib/Data Storage/raptor_data_read  dataName='EPT_EW_STA'  dataShape=Scalar  idxSource=Input  idxRow=1  idxCol=1
      settings: SourceProductName=Raptor
  raptor_data_read3 : Raptor_lib/Data Storage/raptor_data_read  dataName='Flag_Drive_Mode'  dataShape=Scalar  idxSource=Input  idxRow=1  idxCol=1
      settings: SourceProductName=Raptor
  raptor_data_read4 : Raptor_lib/Data Storage/raptor_data_read  dataName='Flag_CHG_Mode'  dataShape=Scalar  idxSource=Input  idxRow=1  idxCol=1
      settings: SourceProductName=Raptor
  raptor_data_read5 : Raptor_lib/Data Storage/raptor_data_read  dataName='Position_R'  dataShape=Scalar  idxSource=Input  idxRow=1  idxCol=1
      settings: SourceProductName=Raptor
  raptor_data_read6 : Raptor_lib/Data Storage/raptor_data_read  dataName='Position_P'  dataShape=Scalar  idxSource=Input  idxRow=1  idxCol=1
      settings: SourceProductName=Raptor
  raptor_data_read7 : Raptor_lib/Data Storage/raptor_data_read  dataName='Position_N'  dataShape=Scalar  idxSource=Input  idxRow=1  idxCol=1
      settings: SourceProductName=Raptor
  raptor_data_read8 : Raptor_lib/Data Storage/raptor_data_read  dataName='Position_D'  dataShape=Scalar  idxSource=Input  idxRow=1  idxCol=1
      settings: SourceProductName=Raptor
  raptor_data_read9 : Raptor_lib/Data Storage/raptor_data_read  dataName='HV_Off'  dataShape=Scalar  idxSource=Input  idxRow=1  idxCol=1
      settings: SourceProductName=Raptor
  raptor_data_write1 : Raptor_lib/Data Storage/raptor_data_write  dataName='LED_Status'  dataShape=Scalar  idxSource=Input Port  idxRow=1  idxCol=1
      settings: SourceProductName=Raptor
  wires:
  raptor_data_read1/1 -> Switch Case/1
  CountTrigger2/1(Tirgger) -> 10Hz/Trigger
  Constant3/1 -> CountTrigger2/1(Counter)
  Constant1/1 -> CountTrigger1/1(Counter)
  CountTrigger1/1(Tirgger) -> 1Hz/Trigger
  CountTrigger3/1(Tirgger) -> 0.5Hz/Trigger
  Constant2/1 -> CountTrigger3/1(Counter)
  CountTrigger4/1(Tirgger) -> 2Hz/Trigger
  Constant4/1 -> CountTrigger4/1(Counter)
  Constant5/1 -> CountTrigger5/1(Counter)
  CountTrigger5/1(Tirgger) -> 4Hz/Trigger
  Switch Case/8 -> Alarrn_LED/Action
  Switch Case/2 -> Charging/Action
  Switch Case/3 -> EVSE Conected/Action
  Switch Case/4 -> P/Action
  Switch Case/5 -> R/Action
  Switch Case/6 -> N/Action
  Switch Case/7 -> "D "/Action
  raptor_adjustment/1 -> CountTrigger6/1(Counter)
  CountTrigger6/1(Tirgger) -> 100Hz/Trigger
  Switch Case/1 -> No Mode/Action
  Constant7/1 -> Switch/1
  raptor_data_read6/1 -> Logical Operator/2
  Logical Operator/1 -> Switch1/2
  Constant8/1 -> Switch1/1
  Logical Operator1/1 -> Switch2/2
  Switch2/1 -> Switch1/3
  Constant9/1 -> Switch2/1
  raptor_data_read5/1 -> Logical Operator1/2
  raptor_data_read7/1 -> Logical Operator2/2
  raptor_data_read8/1 -> Logical Operator3/2
  raptor_data_read3/1 -> NOT/1, Logical Operator2/1, Logical Operator3/1, Logical Operator1/1, Logical Operator/1
  Logical Operator2/1 -> Switch3/2
  Logical Operator3/1 -> Switch4/2
  Constant11/1 -> Switch4/1
  Constant10/1 -> Switch3/1
  Switch3/1 -> Switch2/3
  Switch4/1 -> Switch3/3
  raptor_data_read4/1 -> Switch5/2, NOT1/1
  raptor_data_read2/1 -> Logical Operator4/1
  raptor_data_read9/1 -> Logical Operator4/2
  Logical Operator4/1 -> Switch/2
  Constant12/1 -> Switch5/1
  NOT/1 -> Logical Operator5/1
  NOT1/1 -> Logical Operator5/2
  Logical Operator5/1 -> Switch6/2
  Constant13/1 -> Switch6/1
  Switch5/1 -> Switch6/3
  Switch1/1 -> Switch5/3
  Switch6/1 -> Switch/3
  Switch/1 -> raptor_data_write1/1

== system EPT/Power Up_Down/Background/ Shutdown Event ==
  Trigger : TriggerPort  TriggerType=falling  VariantControl=Variant
  Constant1 : Constant
  Data Type Conversion : DataTypeConversion
  raptor_data_write1 : Raptor_lib/Data Storage/raptor_data_write  dataName='Flag_PowerOff_Finished'  dataShape=Scalar  idxSource=Input Port  idxRow=1  idxCol=1
      settings: SourceProductName=Raptor
  raptor_data_write2 : Raptor_lib/Data Storage/raptor_data_write  dataName='Fault_Reset_Trigger'  dataShape=Scalar  idxSource=Input Port  idxRow=1  idxCol=1
      settings: SourceProductName=Raptor
  raptor_data_write4 : Raptor_lib/Data Storage/raptor_data_write  dataName='Flag_Ign_Off'  dataShape=Scalar  idxSource=Input Port  idxRow=1  idxCol=1
      settings: SourceProductName=Raptor
  wires:
  Constant1/1 -> Data Type Conversion/1
  Data Type Conversion/1 -> raptor_data_write2/1, raptor_data_write1/1, raptor_data_write4/1

== system EPT/Power Up_Down/Background/Debounce ==
  note: Set / Reset
  In : Inport
  Add : Sum
  Constant : Constant  Value=double(0)
  Detect Change : simulink/Logic and Bit Operations/Detect Change  vinit=0  OutDataTypeStr=boolean
  Logic : CombinatorialLogic  TruthTable=[0;1;0;0;1;1;0;0]
  Logical Operator1 : Logic  AllPortsSameDT=off  OutDataTypeStr=boolean
  Logical Operator2 : Logic  AllPortsSameDT=off  OutDataTypeStr=boolean
  Logical Operator3 : Logic  Operator=NOT  Inputs=1  AllPortsSameDT=off  OutDataTypeStr=boolean
  Multiport Switch1 : MultiPortSwitch  DataPortOrder=Zero-based contiguous  Inputs=2  zeroidx=on
  Mux1 : Mux  Inputs=3
  Relational Operator : RelationalOperator  OutDataTypeStr=boolean  RndMeth=Nearest
  Relational Operator1 : RelationalOperator  OutDataTypeStr=boolean  RndMeth=Nearest
  Unit Delay : UnitDelay  SampleTime=-1  HasFrameUpgradeWarning=on
  Unit Delay2 : UnitDelay  InitialCondition=1  SampleTime=-1  HasFrameUpgradeWarning=on
  raptor_adjustment3 : Raptor_lib/Data Storage/raptor_adjustment  paramName='KeySwHiTimeThr'  nameSource=Parameter  initValue=0.2  dataType=double  storage=Calibration  calDispType=Number  calEnum={'Active Low', 'Active High'}  calGain=1  calOffset=0  calMax=inf  calMin=-inf  calFormat='-1'  calUnit='sec'  calHelp='State high time threshold'  calAccess=1  calFunction=group  calDispHeaders=off  calColHeaders={'Col1' 'Col2' 'Col3'}  calRowHeaders={'Row1' 'Row2' 'Row3'}
      settings: SourceProductName=Raptor
  raptor_adjustment4 : Raptor_lib/Data Storage/raptor_adjustment  paramName='KeySwLoTimeThr'  nameSource=Parameter  initValue=0.2  dataType=double  storage=Calibration  calDispType=Number  calEnum={'Active Low', 'Active High'}  calGain=1  calOffset=0  calMax=inf  calMin=-inf  calFormat='-1'  calUnit='sec'  calHelp='State low time threshold'  calAccess=1  calFunction=group  calDispHeaders=off  calColHeaders={'Col1' 'Col2' 'Col3'}  calRowHeaders={'Row1' 'Row2' 'Row3'}
      settings: SourceProductName=Raptor
  raptor_delta_time : Raptor_lib/Triggers/raptor_delta_time  unit=seconds
      settings: SourceProductName=Raptor
  Out : Outport  VectorParamsAs1DForOutWhenUnconnected=off
  wires:
  Detect Change/1 -> Multiport Switch1/1
  Logical Operator3/1 -> Logical Operator2/1
  Relational Operator/1 -> Logical Operator1/2
  Logical Operator2/1 -> Mux1/2
  Logical Operator1/1 -> Mux1/1
  Mux1/1 -> Logic/1
  Unit Delay2/1 -> Mux1/3
  In/1 -> Detect Change/1, Logical Operator1/1, Logical Operator3/1
  Multiport Switch1/1 -> Unit Delay/1, Relational Operator/1, Relational Operator1/1
  Add/1 -> Multiport Switch1/2
  Constant/1 -> Multiport Switch1/3
  Relational Operator1/1 -> Logical Operator2/2
  Logic/1 -> Unit Delay2/1, Out/1
  Unit Delay/1 -> Add/2
  raptor_delta_time/1 -> Add/1
  raptor_adjustment4/1 -> Relational Operator1/2
  raptor_adjustment3/1 -> Relational Operator/2

== system EPT/Power Up_Down/Background/Raise Shutdown Event ==
  Trigger : TriggerPort  TriggerType=falling  VariantControl=Variant
  Constant : Constant  Value=boolean(1)
  Function-Call Generator : simulink/Ports & Subsystems/Function-Call Generator  sample_time=-1  numberOfIterations=1
  raptor_data_def : Raptor_lib/Data Storage/raptor_data_def  dataName='FgndTasksStopped'  initValue=0  dataType=boolean  storage=Volatile (RAM)  calVisible=on  calType=Measurement  calDispType=Number  calEnum={'False', 'True'}  calGain=1.0  calOffset=0  calMin=-Inf  calMax=Inf  calFormat='-1'  calUnit='Bool'  calHelp='Boolean indicating foreground tasks stopped'  calAccess=1  calFunction=group  calDispHeaders=off  calColHeaders={'Col1' 'Col2' 'Col3'}  calRowHeaders={'Row1' 'Row2' 'Row3'}
      settings: SourceProductName=Raptor
  raptor_data_write : Raptor_lib/Data Storage/raptor_data_write  dataName='FgndTasksStopped'  dataShape=Scalar  idxSource=Input Port  idxRow=1  idxCol=1
      settings: SourceProductName=Raptor
  raptor_shutdown : Raptor_lib/Triggers/raptor_shutdown  null=0
      settings: SourceProductName=Raptor
  wires:
  Constant/1 -> raptor_data_write/1
  Function-Call Generator/1 -> raptor_shutdown/Trigger

== system EPT/Power Up_Down/Background/Raise Startup Event ==
  Enable : EnablePort
  Trigger : TriggerPort  VariantControl=Variant
  Function-Call Generator : simulink/Ports & Subsystems/Function-Call Generator  sample_time=-1  numberOfIterations=1
  raptor_startup : Raptor_lib/Triggers/raptor_startup  null=0
      settings: SourceProductName=Raptor
  wires:
  Function-Call Generator/1 -> raptor_startup/Trigger

== system EPT/Power Up_Down/Background/Store EEPROM ==
  Trigger : TriggerPort  TriggerType=falling  VariantControl=Variant
  Function-Call Generator : simulink/Ports & Subsystems/Function-Call Generator  sample_time=-1  numberOfIterations=1
  raptor_store_nv : Raptor_lib/Data Storage/raptor_store_nv  null=0
      settings: SourceProductName=Raptor
  wires:
  Function-Call Generator/1 -> raptor_store_nv/Trigger

== system EPT/Power Up_Down/Background/Store EEPROM Value ==
  Trigger : TriggerPort  TriggerType=falling  VariantControl=Variant
  Relational Operator{,1..3} (4 alike) : RelationalOperator  Operator=~=  OutDataTypeStr=boolean  RndMeth=Simplest
  Subsystem : Subsystem
  Subsystem1 : Subsystem
  Subsystem2 : Subsystem
  Subsystem3 : Subsystem
  raptor_data_read : Raptor_lib/Data Storage/raptor_data_read  dataName='EPT_BPOBU_RCAP'  dataShape=Scalar  idxSource=Input  idxRow=1  idxCol=1
      settings: SourceProductName=Raptor
  raptor_data_read1 : Raptor_lib/Data Storage/raptor_data_read  dataName='EEPROM_RCAP'  dataShape=Scalar  idxSource=Input  idxRow=1  idxCol=1
      settings: SourceProductName=Raptor
  raptor_data_read2 : Raptor_lib/Data Storage/raptor_data_read  dataName='DOD_t'  dataShape=Scalar  idxSource=Input  idxRow=1  idxCol=1
      settings: SourceProductName=Raptor
  raptor_data_read3 : Raptor_lib/Data Storage/raptor_data_read  dataName='EEPROM_DOD_t0'  dataShape=Scalar  idxSource=Input  idxRow=1  idxCol=1
      settings: SourceProductName=Raptor
  raptor_data_read4 : Raptor_lib/Data Storage/raptor_data_read  dataName='EEPROM_SOH'  dataShape=Scalar  idxSource=Input  idxRow=1  idxCol=1
      settings: SourceProductName=Raptor
  raptor_data_read5 : Raptor_lib/Data Storage/raptor_data_read  dataName='New_SOH'  dataShape=Scalar  idxSource=Input  idxRow=1  idxCol=1
      settings: SourceProductName=Raptor
  raptor_data_read6 : Raptor_lib/Data Storage/raptor_data_read  dataName='EPT_BPOBU_FCCAP'  dataShape=Scalar  idxSource=Input  idxRow=1  idxCol=1
      settings: SourceProductName=Raptor
  raptor_data_read7 : Raptor_lib/Data Storage/raptor_data_read  dataName='EEPROM_FCCAP'  dataShape=Scalar  idxSource=Input  idxRow=1  idxCol=1
      settings: SourceProductName=Raptor
  raptor_nv_startup : Raptor_lib/Data Storage/raptor_nv_startup  redundant=off  nv_startup=Keep Saved Values  nv_startup_access=1  redundant_fixed=off  fnv_startup=Keep Saved  fnv_startup_access=1  showRedundant=true  showFixed=true
      settings: SourceProductName=Raptor
  wires:
  Relational Operator/1 -> Subsystem/Enable
  raptor_data_read1/1 -> Relational Operator/2
  raptor_data_read/1 -> Relational Operator/1
  raptor_data_read2/1 -> Relational Operator1/1
  raptor_data_read3/1 -> Relational Operator1/2
  Relational Operator1/1 -> Subsystem1/Enable
  Relational Operator2/1 -> Subsystem2/Enable
  raptor_data_read4/1 -> Relational Operator2/1
  raptor_data_read5/1 -> Relational Operator2/2
  Relational Operator3/1 -> Subsystem3/Enable
  raptor_data_read7/1 -> Relational Operator3/1
  raptor_data_read6/1 -> Relational Operator3/2

== system EPT/Test/Coulomb Counting Method Test/5ms ==
  note: Ampere input
  note: Ah Output
  Enable : EnablePort
  Add1 : Sum
  Add2 : Sum
  Add3 : Sum
  Constant1 : Constant  Value=60
  Constant2 : Constant  Value=200
  Constant3 : Constant  Value=200
  Constant4 : Constant  Value=60
  CountTrigger3 : Subsystem
  CountTrigger4 : Subsystem
  Delay1 : Delay  DelayLength=1  InitialCondition=0
  Delay10 : Delay  DelayLength=1  InitialCondition=0
  Delay2 : Delay  DelayLength=1  InitialCondition=0
  Divide1 : Product  Inputs=*/
  Divide2 : Product  Inputs=*/
  Divide3 : Product  Inputs=*/
  Gain4 : Gain  Gain=60
  Switch{1..2,6,8} (4 alike) : Switch  Criteria=u2 > Threshold
  Output2 : Outport  VectorParamsAs1DForOutWhenUnconnected=off
  wires:
  Delay10/1 -> Add1/2
  CountTrigger4/1(Tirgger) -> Switch6/2, Switch8/2
  Gain4/1 -> CountTrigger4/1(Counter)
  Switch6/1 -> Delay10/1
  Add1/1 -> Switch6/3, Switch8/1
  Switch8/1 -> Divide2/1
  Constant4/1 -> Divide1/2
  Divide1/1 -> Add1/1
  Constant1/1 -> Divide2/2
  CountTrigger3/1(Tirgger) -> Switch1/2, Switch2/2
  Add2/1 -> Switch2/1, Switch1/3
  Switch1/1 -> Delay1/1
  Delay1/1 -> Add2/2
  Switch2/1 -> Divide1/1
  Delay2/1 -> Add3/2
  Add3/1 -> Output2/1, Delay2/1
  Divide2/1 -> Add3/1
  Constant3/1 -> Gain4/1, Divide3/2, CountTrigger3/1(Counter)
  Divide3/1 -> Add2/1
  Constant2/1 -> Divide3/1

== system EPT/Test/Coulomb Counting Method Test/CountTrigger ==
  Counter : Inport
  Constant1 : Constant  Value=0
  Constant3 : Constant
  CycleTrigger : Subsystem
  Switch : Switch  Threshold=1
  Unit Delay1 : UnitDelay  SampleTime=-1  HasFrameUpgradeWarning=on
  Unit Delay2 : UnitDelay  SampleTime=-1  HasFrameUpgradeWarning=on
  Tirgger : Outport  VectorParamsAs1DForOutWhenUnconnected=off
  wires:
  Switch/1 -> Unit Delay1/1
  Constant3/1 -> Switch/3
  Constant1/1 -> Switch/1
  Counter/1 -> CycleTrigger/2(In2)
  CycleTrigger/1(Trigger) -> Switch/2, Unit Delay2/1
  Unit Delay1/1 -> CycleTrigger/1(In1)
  Unit Delay2/1 -> Tirgger/1

== system EPT/Test/DualLEDTest/GreenBreath ==
  Action Port : ActionPort
  Add1 : Sum
  Compare To Constant2 : simulink/Logic and Bit Operations/Compare To Constant  relop=<  const=0  OutDataTypeStr=boolean
  Compare To Constant3 : simulink/Logic and Bit Operations/Compare To Constant  relop=>  const=10000  OutDataTypeStr=boolean
  Constant5 : Constant  Value=50
  Data Type Conversion : DataTypeConversion
  Data Type Conversion1 : DataTypeConversion
  Gain2 : Gain  Gain=-1
  If : If  IfExpression=u1 >= 1  ShowElse=off
  Logical Operator1 : Logic  Operator=OR  AllPortsSameDT=off  OutDataTypeStr=boolean
  Scope1 : Scope
  Scope2 : Scope
  Switch : Switch  Threshold=1
  Transition state : Subsystem  TreatAsAtomicUnit=on
  Unit Delay : UnitDelay  SampleTime=-1  HasFrameUpgradeWarning=on
  raptor_data_read : Raptor_lib/Data Storage/raptor_data_read  dataName='LED_Gradient'  dataShape=Scalar  idxSource=Input  idxRow=1  idxCol=1
      settings: SourceProductName=Raptor
  raptor_data_write : Raptor_lib/Data Storage/raptor_data_write  dataName='LED_Duty'  dataShape=Scalar  idxSource=Input Port  idxRow=1  idxCol=1
      settings: SourceProductName=Raptor
  wires:
  Gain2/1 -> Switch/1
  Constant5/1 -> Gain2/1, Switch/3
  If/1 -> Transition state/Action
  Logical Operator1/1 -> Data Type Conversion1/1
  Compare To Constant2/1 -> Logical Operator1/1
  Compare To Constant3/1 -> Logical Operator1/2
  Data Type Conversion1/1 -> If/1
  Data Type Conversion/1 -> raptor_data_write/1, Scope2/1
  raptor_data_read/1 -> Switch/2
  Unit Delay/1 -> Add1/1
  Add1/1 -> Compare To Constant3/1, Compare To Constant2/1, Scope1/1, Unit Delay/1, Data Type Conversion/1
  Switch/1 -> Add1/2

== system EPT/Test/DualLEDTest/RedBreath ==
  Action Port : ActionPort
  Add1 : Sum
  Compare To Constant : simulink/Logic and Bit Operations/Compare To Constant  relop=>  const=0  OutDataTypeStr=boolean
  Compare To Constant1 : simulink/Logic and Bit Operations/Compare To Constant  relop=<  const=-10000  OutDataTypeStr=boolean
  Constant5 : Constant  Value=50
  Data Type Conversion : DataTypeConversion
  Data Type Conversion1 : DataTypeConversion
  Gain2 : Gain  Gain=-1
  If : If  IfExpression=u1 >= 1  ShowElse=off
  Logical Operator : Logic  Operator=OR  AllPortsSameDT=off  OutDataTypeStr=boolean
  Scope1 : Scope
  Scope2 : Scope
  Switch : Switch  Threshold=1
  Transition state : Subsystem  TreatAsAtomicUnit=on
  Unit Delay : UnitDelay  SampleTime=-1  HasFrameUpgradeWarning=on
  raptor_data_read : Raptor_lib/Data Storage/raptor_data_read  dataName='LED_Gradient'  dataShape=Scalar  idxSource=Input  idxRow=1  idxCol=1
      settings: SourceProductName=Raptor
  raptor_data_write : Raptor_lib/Data Storage/raptor_data_write  dataName='LED_Duty'  dataShape=Scalar  idxSource=Input Port  idxRow=1  idxCol=1
      settings: SourceProductName=Raptor
  wires:
  Gain2/1 -> Switch/1
  Constant5/1 -> Gain2/1, Switch/3
  Data Type Conversion1/1 -> If/1
  If/1 -> Transition state/Action
  Data Type Conversion/1 -> raptor_data_write/1, Scope2/1
  raptor_data_read/1 -> Switch/2
  Compare To Constant/1 -> Logical Operator/1
  Unit Delay/1 -> Add1/1
  Add1/1 -> Compare To Constant/1, Compare To Constant1/1, Scope1/1, Unit Delay/1, Data Type Conversion/1
  Switch/1 -> Add1/2
  Logical Operator/1 -> Data Type Conversion1/1
  Compare To Constant1/1 -> Logical Operator/2

== system EPT/Test/LED For CMU/CMU_Fault  ==
  Action Port : ActionPort
  Constant1 : Constant  Value=6000
  Data Type Conversion : DataTypeConversion
  raptor_data_write : Raptor_lib/Data Storage/raptor_data_write  dataName='LED_Duty'  dataShape=Scalar  idxSource=Input Port  idxRow=1  idxCol=1
      settings: SourceProductName=Raptor
  wires:
  Data Type Conversion/1 -> raptor_data_write/1
  Constant1/1 -> Data Type Conversion/1

== system EPT/Test/LED For CMU/CMU_NotWork ==
  Action Port : ActionPort
  Constant1 : Constant  Value=0
  Data Type Conversion : DataTypeConversion
  raptor_data_write : Raptor_lib/Data Storage/raptor_data_write  dataName='LED_Duty'  dataShape=Scalar  idxSource=Input Port  idxRow=1  idxCol=1
      settings: SourceProductName=Raptor
  wires:
  Constant1/1 -> Data Type Conversion/1
  Data Type Conversion/1 -> raptor_data_write/1

== system EPT/Test/LED For CMU/CMU_Ok ==
  Action Port : ActionPort
  Constant1 : Constant  Value=-6000
  Data Type Conversion : DataTypeConversion
  raptor_data_write : Raptor_lib/Data Storage/raptor_data_write  dataName='LED_Duty'  dataShape=Scalar  idxSource=Input Port  idxRow=1  idxCol=1
      settings: SourceProductName=Raptor
  wires:
  Data Type Conversion/1 -> raptor_data_write/1
  Constant1/1 -> Data Type Conversion/1

== system EPT/Test/LED For CMU/Latch2 ==
  Latch : Inport
  Reset : Inport  Port=2
  Switch1 : Switch  Criteria=u2 > Threshold
  Switch3 : Switch  Criteria=u2 > Threshold
  Unit Delay1 : UnitDelay  SampleTime=-1  HasFrameUpgradeWarning=on
  Output : Outport  VectorParamsAs1DForOutWhenUnconnected=off
  wires:
  Unit Delay1/1 -> Switch1/3
  Switch3/1 -> Output/1, Unit Delay1/1
  Reset/1 -> Switch3/2
  Latch/1 -> Switch1/1, Switch1/2
  Switch1/1 -> Switch3/3

== system EPT/Test/LED For CMU/deBounce 2 ==
  >= : Inport
  TimeCount1 : Inport  Port=2
  Constant10 : Constant
  Constant11 : Constant  Value=0
  Constant8 : Constant  Value=0
  CycleTrigger1 : Subsystem
  Switch2 : Switch  Threshold=1
  Switch3 : Switch  Threshold=1
  Unit Delay2 : UnitDelay  SampleTime=-1  HasFrameUpgradeWarning=on
  Tirgger1 : Outport  VectorParamsAs1DForOutWhenUnconnected=off
  wires:
  Constant11/1 -> Switch3/3
  Switch2/1 -> Switch3/1
  Switch3/1 -> CycleTrigger1/1(In1)
  Constant10/1 -> Switch2/3
  Unit Delay2/1 -> Switch2/2
  Constant8/1 -> Switch2/1
  CycleTrigger1/1(Trigger) -> Tirgger1/1, Unit Delay2/1
  >=/1 -> Switch3/2
  TimeCount1/1 -> CycleTrigger1/2(In2)

== system EPT/Test/LifeCycleTest/LifeCycleDetect ==
  LifeCycle : Inport
  DataIn : Inport  Port=2
  Reset : Inport  Port=3
  Add1 : Sum
  Constant1 : Constant  Value=5
  Constant2 : Constant
  Delay1 : Delay  DelayLength=1  InitialCondition=0
  Delay2 : Delay  DelayLength=1  InitialCondition=0
  Detect Change : simulink/Logic and Bit Operations/Detect Change  vinit=0  OutDataTypeStr=boolean
  Latch1 : Subsystem
  Relational Operator : RelationalOperator  Operator=>  OutDataTypeStr=boolean  RndMeth=Simplest
  Switch3 : Switch  Criteria=u2 > Threshold
  Switch4 : Switch  Criteria=u2 > Threshold
  DataOut : Outport  VectorParamsAs1DForOutWhenUnconnected=off
  Trigger : Outport  Port=2  VectorParamsAs1DForOutWhenUnconnected=off
  wires:
  Detect Change/1 -> Switch4/2, Switch3/2
  Constant2/1 -> Add1/1
  Switch3/1 -> DataOut/1, Delay2/1
  Switch4/1 -> Relational Operator/1, Delay1/1
  Add1/1 -> Switch4/3
  LifeCycle/1 -> Detect Change/1
  Delay2/1 -> Switch3/3
  Delay1/1 -> Add1/2
  Relational Operator/1 -> Latch1/1(Latch)
  DataIn/1 -> Switch3/1
  Latch1/1(Output) -> Trigger/1
  Constant1/1 -> Relational Operator/2
  Reset/1 -> Latch1/2(Reset)
